simulink model "Australian14gen_R2017a"  (R2017a)
settings: Solver=ode23tb  StartTime=0.0  StopTime=50  FixedStep=1/50  MaxStep=1/50  RelTol=1e-3  AbsTol=1e-1  EnableMultiTasking=on
PreLoadFcn:
  | dataaustralian14gen
values from neighbouring files (symbols this model uses):
  bus_v = [ 101	15 ... (first row only)    [dataaustralian14gen.m]
  comp = [ 1	211	0	0 ... (first row only)    [dataaustralian14gen.m]
  Exc = [ 101	0	 200	0.1	    13.25  2.5	 0	0       0       0       0       0 ... (first row only)    [dataaustralian14gen.m]
  FH = 13    [dataaustralian14gen.m]
  FI = 1    [dataaustralian14gen.m]
  FL = .1    (= 0.1)    [dataaustralian14gen.m]
  G_data = [ 101	333.3	15	3.6	0.14	1.1	0.65	0.25	8.5     0.20	0.05	0       0       0.25	0.2 	0 ... (first row only)    [dataaustralian14gen.m]
  KH = 120    [dataaustralian14gen.m]
  KI = 10    [dataaustralian14gen.m]
  KL = 10    [dataaustralian14gen.m]
  line = [ 102	217	0.0084	0.0667	0.817	330	1 ... (first row only)    [dataaustralian14gen.m]
  p = p_case1    [dataaustralian14gen.m]
  PSSMODEL = 1    [dataaustralian14gen.m]
  SVC = [ 205	650 430   -220 1.055  -68.3 ... (first row only)    [dataaustralian14gen.m]
  trans = [     1   101   102    15   330   333.3    12     12    0.9390 ... (first row only)    [dataaustralian14gen.m]
undefined symbols (not defined in the file or in its folder): D1, Delta
libraries: powerlib x371, sps_avr x14, powerlib_extras x9, factslib x5
(part 2 of 3)

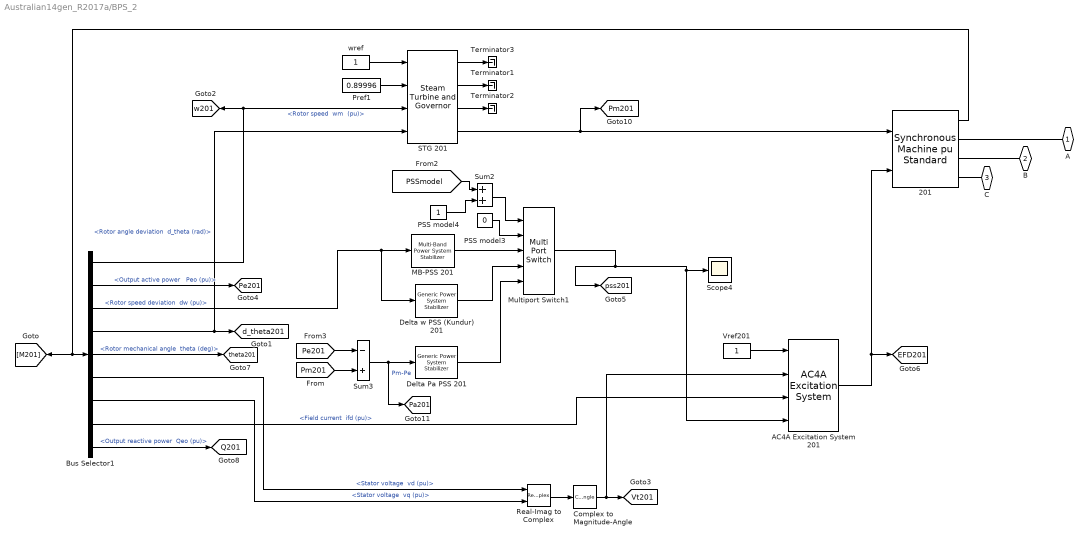
== system Australian14gen_R2017a/BPS_2 ==
  201 : powerlib/Machines/Synchronous Machine pu Standard  PresetModel=No  MechanicalLoad=Mechanical power Pm  ShowDetailedParameters=on  RotorType=Round  Units=per unit standard parameters  MeasurementBus=off  NominalParameters="[G_data(2,2)*1e6  G_data(2,3)*1e3  50]"  Reactances1=[G_data(2,6),G_data(2,8),G_data(2,10),G_data(2,7),G_data(2,12),G_data(2,14),G_data(2,5)]  Reactances2=[G_data(2,6),G_data(2,8),G_data(2,10),G_data(2,7),G_data(2,14),G_data(2,5)]  dAxisTimeConstants=Open-circuit  qAxisTimeConstants=Open-circuit  TimeConstants1="[G_data(2,9)  G_data(2,11)  G_data(2,15)]"  TimeConstants2="[G_data(2,9), G_data(2,11), G_data(2,13),  G_data(2,15)]"  TimeConstants3="[  5.9  0.033  0.023  ]"  TimeConstants4=[ 8.0, 0.03, 0.3371, 0.0295 ]  TimeConstants5=[ 1.01, 0.053, 0.1 ]  TimeConstants6=[ 1.3201, 0.023, 1.0, 0.07 ]  TimeConstants7="[  1.01  0.053  0.051266  ]"  TimeConstants8=[ 1.3201, 0.0231, 0.3371, 0.0295 ]  StatorResistance=0  Mechanical="[ G_data(2,4) 0  4 ]"  PolePairs=4  InitialConditions=[0 9.38697 0.909099 0.909099 0.909099 39.1318 -80.8682 159.132 2.03476]  SetSaturation=off  Saturation=[0.6404,0.7127,0.8441,0.9214,0.9956,1.082,1.19,1.316,1.457;0.7,0.7698,0.8872,0.9466,0.9969,1.046,1.1,1.151,1.201]  LoadFlowParameters=[1 3600000000 20000 0 0]  TsPowergui=0  TsBlock=-1  IterativeModel=Forward Euler  IterativeDiscreteModel=Trapezoidal non iterative  BusType=PV  Pref=p(2,3)*1e6  Qref=0  Qmin=-inf  Qmax=inf  PLF=0  QLF=0
      settings: SourceProductName=Simscape Power Systems
  AC4A Excitation System 201 : sps_avr/AC4A Excitation System  Tr=Exc(2,2)  KaTa="[Exc(2,3)   Exc(2,4)]"  VIminmax=[-10 10]  VRminmax=[-4.53 5.64]  TbTc="[Exc(2,5)  Exc(2,6)]"  Kc=0  v0=[1 2.0348]  TsBlock=0
      settings: SourceProductName=Simscape Power Systems  SourceProductBaseCode=PS
  Bus Selector1 : BusSelector  OutputSignals="Mechanical.Rotor speed  wm  (pu),Output active power   Peo (pu),Mechanical.Rotor speed deviation  dw (pu),Mechanical.Rotor angle deviation  d_theta (rad),Mechanical.Rotor mechanical angle  theta (deg),dq0 components.Stator voltage  vd (pu),dq0 components.Stator voltage  vq (pu),dq0 components.Field current  ifd (pu),Output reactive power  Qeo (pu)"
  Complex to Magnitude-Angle : ComplexToMagnitudeAngle  Output=Magnitude
  Delta Pa PSS 201 : powerlib/Machines/Generic Power System Stabilizer  Tsensor=15e-3  K=2.5*1.25  Twashout=1  Tleadlag1=[60e-3 1]  Tleadlag2=[0 0]  VSlimits=[-0.15 0.15]  Vinit=0  Plot_On=off  MagdB_On=on  FreqRange=logspace(-2,2,500)
      settings: SourceProductName=Simscape Power Systems  SourceProductBaseCode=PS
  Delta w PSS (Kundur) 201 : powerlib/Machines/Generic Power System Stabilizer  Tsensor=15e-3  K=30  Twashout=10  Tleadlag1=[50e-3 20e-3]  Tleadlag2=[3 5.4]  VSlimits=[-0.15 0.15]  Vinit=0  Plot_On=off  MagdB_On=on  FreqRange=logspace(-2,2,500)
      settings: SourceProductName=Simscape Power Systems  SourceProductBaseCode=PS
  MB-PSS 201 : powerlib/Machines/Multi-Band Power System Stabilizer  OperationMode=Simplified settings  Kg=G  GL="[FL  KL]"  GI="[FI  KI]"  GH="[FH  KH]"  GLd=[66 66 9.4]  TcLF=[1.667 2 0 0 0 0 2 2.4 0 0 0 0 1 1]  GId=[66 66 47.6]  TcIF=[1 1 0.25 0.3 0 0 1 1 0.3 0.36 0 0 0 0]  GHd=[66 66 233]  TcHF="[0.01 0.012 0 0 0 0  0.012 0.0144 0 0 0 0 1 1]"  LIM=[.075 .15 .15 .15]  Plot_On=off  MagdB_On=off  FreqRange=logspace(-2,2,500)
      settings: SourceProductName=Simscape Power Systems  SourceProductBaseCode=PS
  Multiport Switch1 : MultiPortSwitch  Inputs=4  InputSameDT=on
  PSS model3 : Constant  Value=0
  PSS model4 : Constant
  Pref1 : Constant  Value=0.89996
  Real-Imag to Complex : RealImagToComplex
  STG 201 : powerlib/Machines/Steam Turbine and Governor  gentype=Tandem-compound (single mass)  reg1="[ 1  0.05    0 ]"  reg2="[ 0.001  0.15 ]"  reg3="[ -0.1  0.1  0  4.496 ]"  N=3000  turb1="[ 0  10   3.3   0.5   ]"  turb2="[   0   0.36    0.36   0.28   ]"  HA="[ 0.046  1.430  1.465   0.192 ]"  KA="[ 90.44  53.88  64.59   62.94  ]"  DA="[ 0.0115  0.3575  0.3663   0.0137  ]"  ini1=0.89996  ini2=[0.779316,-31.4247]
      settings: SourceProductName=Simscape Power Systems  SourceProductBaseCode=PS
  Scope4 : Scope
  Sum2 : Sum  SaturateOnIntegerOverflow=on  InputSameDT=on  OutDataTypeStr=Inherit: Same as first input
  Sum3 : Sum  Inputs=-+  SaturateOnIntegerOverflow=on  InputSameDT=on  OutDataTypeStr=Inherit: Same as first input
  Terminator1 : Terminator
  Terminator2 : Terminator
  Terminator3 : Terminator
  Vref201 : Constant
  wref : Constant
  A : PMIOPort  Port=1  Side=Left
  B : PMIOPort  Port=2  Side=Left
  C : PMIOPort  Port=3  Side=Left
  tag scope: EFD201=global, Pa201=global, Pe201=global, Pm201=global, Q201=global, Vt201=global, d_theta201=global, pss201=global, theta201=global, w201=global
  wires:
  Bus Selector1/7 -> Real-Imag to Complex/2  "<Stator voltage  vq (pu)>"
  Bus Selector1/6 -> Real-Imag to Complex/1  "<Stator voltage  vd (pu)>"
  wref/1 -> STG 201/1
  Vref201/1 -> AC4A Excitation System 201/1
  Bus Selector1/4 -> STG 201/4, [d_theta201]  "<Rotor angle deviation  d_theta (rad)>"
  201/1 -> Bus Selector1/1, [M201]
  Bus Selector1/1 -> [w201], STG 201/3  "<Rotor speed  wm  (pu)>"
  Bus Selector1/3 -> Delta w PSS (Kundur) 201/1, MB-PSS 201/1  "<Rotor speed deviation  dw (pu)>"
  Real-Imag to Complex/1 -> Complex to Magnitude-Angle/1
  Complex to Magnitude-Angle/1 -> AC4A Excitation System 201/2, [Vt201]
  AC4A Excitation System 201/1 -> 201/2, [EFD201]
  Bus Selector1/5 -> [theta201]  "<Rotor mechanical angle  theta (deg)>"
  Bus Selector1/2 -> [Pe201]  "<Output active power   Peo (pu)>"
  Bus Selector1/8 -> AC4A Excitation System 201/3  "<Field current  ifd (pu)>"
  STG 201/4 -> 201/1, [Pm201]
  Bus Selector1/9 -> [Q201]  "<Output reactive power  Qeo (pu)>"
  PSS model4/1 -> Sum2/2
  Sum2/1 -> Multiport Switch1/1
  [PSSmodel] -> Sum2/1
  PSS model3/1 -> Multiport Switch1/2
  Sum3/1 -> [Pa201], Delta Pa PSS 201/1  "Pm-Pe"
  Delta Pa PSS 201/1 -> Multiport Switch1/5
  Delta w PSS (Kundur) 201/1 -> Multiport Switch1/4
  [Pm201] -> Sum3/2
  [Pe201] -> Sum3/1
  MB-PSS 201/1 -> Multiport Switch1/3
  STG 201/1 -> Terminator3/1
  STG 201/2 -> Terminator1/1
  STG 201/3 -> Terminator2/1
  Pref1/1 -> STG 201/2
  Multiport Switch1/1 -> Scope4/1, AC4A Excitation System 201/4, [pss201]
  connections:
  201/RConn1 -- A/RConn1
  201/RConn2 -- B/RConn1
  201/RConn3 -- C/RConn1

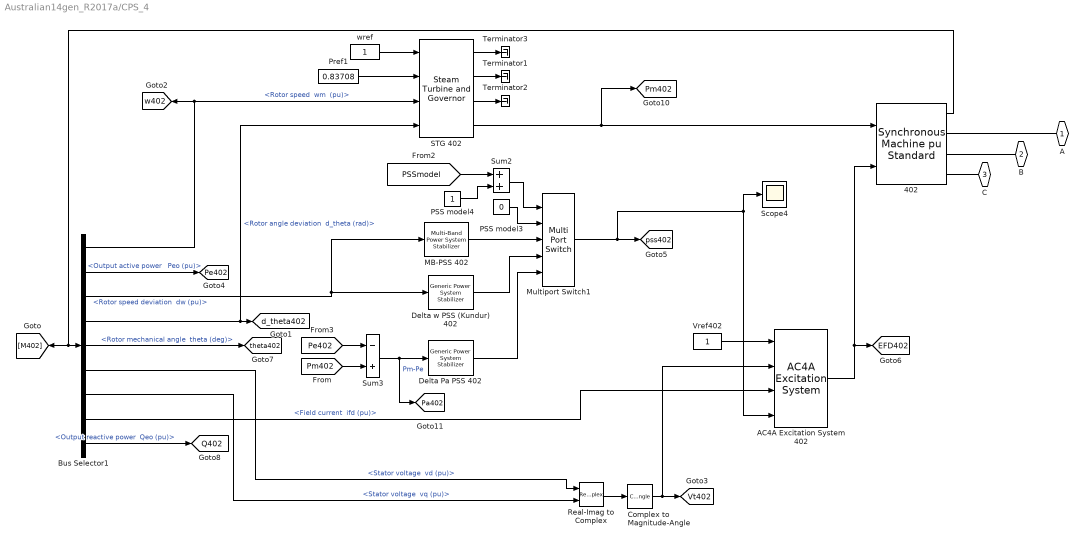
== system Australian14gen_R2017a/CPS_4 ==
  402 : powerlib/Machines/Synchronous Machine pu Standard  PresetModel=No  MechanicalLoad=Mechanical power Pm  ShowDetailedParameters=on  RotorType=Round  Units=per unit standard parameters  MeasurementBus=off  NominalParameters="[G_data(9,2)*1e6  G_data(9,3)*1e3  50]"  Reactances1=[G_data(9,6),G_data(9,8),G_data(9,10),G_data(9,7),G_data(9,12),G_data(9,14),G_data(9,5)]  Reactances2=[G_data(9,6),G_data(9,8),G_data(9,10),G_data(9,7),G_data(9,14),G_data(9,5)]  dAxisTimeConstants=Open-circuit  qAxisTimeConstants=Open-circuit  TimeConstants1="[G_data(9,9)  G_data(9,11)  G_data(9,15)]"  TimeConstants2="[G_data(9,9)  G_data(9,11)  G_data(9,13)  G_data(9,15)]"  TimeConstants3="[  5.9  0.033  0.023  ]"  TimeConstants4=[ 8.0, 0.03, 0.3371, 0.0295 ]  TimeConstants5=[ 1.01, 0.053, 0.1 ]  TimeConstants6=[ 1.3201, 0.023, 1.0, 0.07 ]  TimeConstants7="[  1.01  0.053  0.051266  ]"  TimeConstants8=[ 1.3201, 0.0231, 0.3371, 0.0295 ]  StatorResistance=0  Mechanical="[ G_data(9,4) 0  4 ]"  PolePairs=4  InitialConditions=[0 62.5752 0.854876 0.854876 0.854876 91.9195 -28.0805 211.92 2.07263]  SetSaturation=off  Saturation=[0.6404,0.7127,0.8441,0.9214,0.9956,1.082,1.19,1.316,1.457;0.7,0.7698,0.8872,0.9466,0.9969,1.046,1.1,1.151,1.201]  LoadFlowParameters=[1 837000000 20000 0 0]  TsPowergui=0  TsBlock=-1  IterativeModel=Forward Euler  IterativeDiscreteModel=Trapezoidal non iterative  BusType=PV  Pref=p(9,3)*1e6  Qref=0  Qmin=-inf  Qmax=inf  PLF=0  QLF=0
      settings: SourceProductName=Simscape Power Systems
  AC4A Excitation System 402 : sps_avr/AC4A Excitation System  Tr=Exc(9,2)  KaTa="[Exc(9,3)   Exc(9,4)]"  VIminmax=[-10 10]  VRminmax=[-4.53 5.64]  TbTc="[Exc(9,5)  Exc(9,6)]"  Kc=0  v0=[1 2.0726]  TsBlock=0
      settings: SourceProductName=Simscape Power Systems  SourceProductBaseCode=PS
  Bus Selector1 : BusSelector  OutputSignals="Mechanical.Rotor speed  wm  (pu),Output active power   Peo (pu),Mechanical.Rotor speed deviation  dw (pu),Mechanical.Rotor angle deviation  d_theta (rad),Mechanical.Rotor mechanical angle  theta (deg),dq0 components.Stator voltage  vd (pu),dq0 components.Stator voltage  vq (pu),dq0 components.Field current  ifd (pu),Output reactive power  Qeo (pu)"
  Complex to Magnitude-Angle : ComplexToMagnitudeAngle  Output=Magnitude
  Delta Pa PSS 402 : powerlib/Machines/Generic Power System Stabilizer  Tsensor=15e-3  K=2.5*1.25  Twashout=1  Tleadlag1=[60e-3 1]  Tleadlag2=[0 0]  VSlimits=[-0.15 0.15]  Vinit=0  Plot_On=off  MagdB_On=on  FreqRange=logspace(-2,2,500)
      settings: SourceProductName=Simscape Power Systems  SourceProductBaseCode=PS
  Delta w PSS (Kundur) 402 : powerlib/Machines/Generic Power System Stabilizer  Tsensor=15e-3  K=30  Twashout=10  Tleadlag1=[50e-3 20e-3]  Tleadlag2=[3 5.4]  VSlimits=[-0.15 0.15]  Vinit=0  Plot_On=off  MagdB_On=on  FreqRange=logspace(-2,2,500)
      settings: SourceProductName=Simscape Power Systems  SourceProductBaseCode=PS
  MB-PSS 402 : powerlib/Machines/Multi-Band Power System Stabilizer  OperationMode=Simplified settings  Kg=G  GL="[FL  KL]"  GI="[FI  KI]"  GH="[FH  KH]"  GLd=[66 66 9.4]  TcLF=[1.667 2 0 0 0 0 2 2.4 0 0 0 0 1 1]  GId=[66 66 47.6]  TcIF=[1 1 0.25 0.3 0 0 1 1 0.3 0.36 0 0 0 0]  GHd=[66 66 233]  TcHF="[0.01 0.012 0 0 0 0  0.012 0.0144 0 0 0 0 1 1]"  LIM=[.075 .15 .15 .15]  Plot_On=off  MagdB_On=off  FreqRange=logspace(-2,2,500)
      settings: SourceProductName=Simscape Power Systems  SourceProductBaseCode=PS
  Multiport Switch1 : MultiPortSwitch  Inputs=4  InputSameDT=on
  PSS model3 : Constant  Value=0
  PSS model4 : Constant
  Pref1 : Constant  Value=0.83708
  Real-Imag to Complex : RealImagToComplex
  STG 402 : powerlib/Machines/Steam Turbine and Governor  gentype=Tandem-compound (single mass)  reg1="[ 1  0.05    0 ]"  reg2="[ 0.001  0.15 ]"  reg3="[ -0.1  0.1  0  4.496 ]"  N=3000  turb1="[ 0  10   3.3   0.5   ]"  turb2="[   0   0.36    0.36   0.28   ]"  HA="[ 0.046  1.430  1.465   0.192 ]"  KA="[ 90.44  53.88  64.59   62.94  ]"  DA="[ 0.0115  0.3575  0.3663   0.0137  ]"  ini1=0.83708  ini2=[0.779316,-31.4247]
      settings: SourceProductName=Simscape Power Systems  SourceProductBaseCode=PS
  Scope4 : Scope
  Sum2 : Sum  SaturateOnIntegerOverflow=on  InputSameDT=on  OutDataTypeStr=Inherit: Same as first input
  Sum3 : Sum  Inputs=-+  SaturateOnIntegerOverflow=on  InputSameDT=on  OutDataTypeStr=Inherit: Same as first input
  Terminator1 : Terminator
  Terminator2 : Terminator
  Terminator3 : Terminator
  Vref402 : Constant
  wref : Constant
  A : PMIOPort  Port=1  Side=Left
  B : PMIOPort  Port=2  Side=Left
  C : PMIOPort  Port=3  Side=Left
  tag scope: EFD402=global, Pa402=global, Pe402=global, Pm402=global, Q402=global, Vt402=global, d_theta402=global, pss402=global, theta402=global, w402=global
  wires:
  Bus Selector1/7 -> Real-Imag to Complex/2  "<Stator voltage  vq (pu)>"
  Bus Selector1/6 -> Real-Imag to Complex/1  "<Stator voltage  vd (pu)>"
  wref/1 -> STG 402/1
  Vref402/1 -> AC4A Excitation System 402/1
  Bus Selector1/4 -> STG 402/4, [d_theta402]  "<Rotor angle deviation  d_theta (rad)>"
  402/1 -> Bus Selector1/1, [M402]
  Bus Selector1/1 -> [w402], STG 402/3  "<Rotor speed  wm  (pu)>"
  Bus Selector1/3 -> Delta w PSS (Kundur) 402/1, MB-PSS 402/1  "<Rotor speed deviation  dw (pu)>"
  Real-Imag to Complex/1 -> Complex to Magnitude-Angle/1
  Complex to Magnitude-Angle/1 -> AC4A Excitation System 402/2, [Vt402]
  AC4A Excitation System 402/1 -> 402/2, [EFD402]
  Bus Selector1/5 -> [theta402]  "<Rotor mechanical angle  theta (deg)>"
  Bus Selector1/2 -> [Pe402]  "<Output active power   Peo (pu)>"
  Bus Selector1/8 -> AC4A Excitation System 402/3  "<Field current  ifd (pu)>"
  STG 402/4 -> 402/1, [Pm402]
  Bus Selector1/9 -> [Q402]  "<Output reactive power  Qeo (pu)>"
  PSS model4/1 -> Sum2/2
  Sum2/1 -> Multiport Switch1/1
  [PSSmodel] -> Sum2/1
  PSS model3/1 -> Multiport Switch1/2
  Sum3/1 -> [Pa402], Delta Pa PSS 402/1  "Pm-Pe"
  Delta Pa PSS 402/1 -> Multiport Switch1/5
  Delta w PSS (Kundur) 402/1 -> Multiport Switch1/4
  [Pm402] -> Sum3/2
  [Pe402] -> Sum3/1
  MB-PSS 402/1 -> Multiport Switch1/3
  STG 402/1 -> Terminator3/1
  STG 402/2 -> Terminator1/1
  STG 402/3 -> Terminator2/1
  Pref1/1 -> STG 402/2
  Multiport Switch1/1 -> Scope4/1, AC4A Excitation System 402/4, [pss402]
  connections:
  402/RConn1 -- A/RConn1
  402/RConn2 -- B/RConn1
  402/RConn3 -- C/RConn1

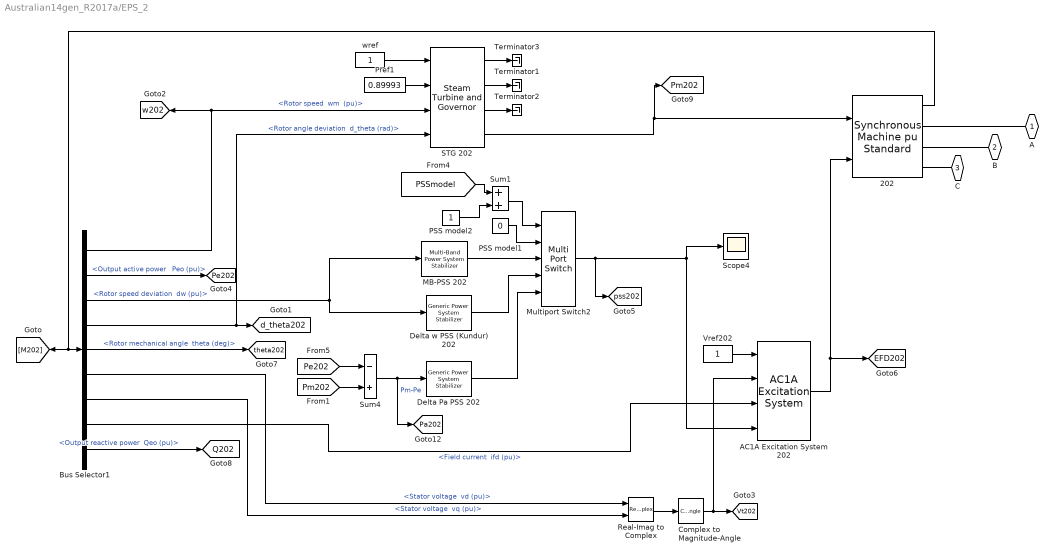
== system Australian14gen_R2017a/EPS_2 ==
  202 : powerlib/Machines/Synchronous Machine pu Standard  PresetModel=No  MechanicalLoad=Mechanical power Pm  ShowDetailedParameters=on  RotorType=Round  Units=per unit standard parameters  MeasurementBus=off  NominalParameters="[G_data(3,2)*1e6  G_data(3,3)*1e3  50]"  Reactances1=[G_data(3,6),G_data(3,8),G_data(3,10),G_data(3,7),G_data(3,12), G_data(3,14),G_data(3,5)]  Reactances2=[G_data(3,6),G_data(3,8),G_data(3,10),G_data(3,7),G_data(3,12), G_data(3,14),G_data(3,5)]  dAxisTimeConstants=Open-circuit  qAxisTimeConstants=Open-circuit  TimeConstants1="[G_data(3,9)  G_data(3,11)  G_data(3,13) G_data(3,15)]"  TimeConstants2="[G_data(3,9)  G_data(3,11)  G_data(3,13) G_data(3,15)]"  TimeConstants3="[  5.9  0.033  0.023  ]"  TimeConstants4=[ 8.0, 0.03, 0.3371, 0.0295 ]  TimeConstants5=[ 1.01, 0.053, 0.1 ]  TimeConstants6=[ 1.3201, 0.023, 1.0, 0.07 ]  TimeConstants7="[  1.01  0.053  0.051266  ]"  TimeConstants8=[ 1.3201, 0.0231, 0.3371, 0.0295 ]  StatorResistance=0  Mechanical="[ G_data(3,4) 0  4 ]"  PolePairs=4  InitialConditions=[0 -1.78632 0.929675 0.929675 0.929675 21.932 -98.068 141.932 2.49164]  SetSaturation=off  Saturation=[0.6404,0.7127,0.8441,0.9214,0.9956,1.082,1.19,1.316,1.457;0.7,0.7698,0.8872,0.9466,0.9969,1.046,1.1,1.151,1.201]  LoadFlowParameters=[1 2500000000 20000 0 0]  TsPowergui=0  TsBlock=-1  IterativeModel=Forward Euler  IterativeDiscreteModel=Trapezoidal non iterative  BusType=PV  Pref=p(3,3)*1e6  Qref=0  Qmin=-inf  Qmax=inf  PLF=0  QLF=0
      settings: SourceProductName=Simscape Power Systems
  AC1A Excitation System 202 : sps_avr/AC1A Excitation System  Tr=Exc(3,2)  KaTa="[Exc(3,3)   Exc(3,4)]"  VAminmax=[-14.5 14.5]  VRminmax=[-5.43 6.03]  KfTf="[Exc(3,9)  Exc(3,10)]"  TbTc="[Exc(3,5)  Exc(3,6)]"  KeTe="[Exc(3,7)  Exc(3,8)]"  Ve12=[4.18 3.14]  SeVe12=[0.10 0.03]  Kd=0.38  Kc=0.20  v0=[1 2.4916]  TsBlock=0
      settings: SourceProductName=Simscape Power Systems  SourceProductBaseCode=PS
  Bus Selector1 : BusSelector  OutputSignals="Mechanical.Rotor speed  wm  (pu),Output active power   Peo (pu),Mechanical.Rotor speed deviation  dw (pu),Mechanical.Rotor angle deviation  d_theta (rad),Mechanical.Rotor mechanical angle  theta (deg),dq0 components.Stator voltage  vd (pu),dq0 components.Stator voltage  vq (pu),dq0 components.Field current  ifd (pu),Output reactive power  Qeo (pu)"
  Complex to Magnitude-Angle : ComplexToMagnitudeAngle  Output=Magnitude
  Delta Pa PSS 202 : powerlib/Machines/Generic Power System Stabilizer  Tsensor=15e-3  K=2.5*1.25  Twashout=1  Tleadlag1=[60e-3 1]  Tleadlag2=[0 0]  VSlimits=[-0.15 0.15]  Vinit=0  Plot_On=off  MagdB_On=on  FreqRange=logspace(-2,2,500)
      settings: SourceProductName=Simscape Power Systems  SourceProductBaseCode=PS
  Delta w PSS (Kundur) 202 : powerlib/Machines/Generic Power System Stabilizer  Tsensor=15e-3  K=30  Twashout=10  Tleadlag1=[50e-3 20e-3]  Tleadlag2=[3 5.4]  VSlimits=[-0.15 0.15]  Vinit=0  Plot_On=off  MagdB_On=on  FreqRange=logspace(-2,2,500)
      settings: SourceProductName=Simscape Power Systems  SourceProductBaseCode=PS
  MB-PSS 202 : powerlib/Machines/Multi-Band Power System Stabilizer  OperationMode=Simplified settings  Kg=G  GL="[FL  KL]"  GI="[FI  KI]"  GH="[FH  KH]"  GLd=[66 66 9.4]  TcLF=[1.667 2 0 0 0 0 2 2.4 0 0 0 0 1 1]  GId=[66 66 47.6]  TcIF=[1 1 0.25 0.3 0 0 1 1 0.3 0.36 0 0 0 0]  GHd=[66 66 233]  TcHF="[0.01 0.012 0 0 0 0  0.012 0.0144 0 0 0 0 1 1]"  LIM=[.075 .15 .15 .15]  Plot_On=off  MagdB_On=off  FreqRange=logspace(-2,2,500)
      settings: SourceProductName=Simscape Power Systems  SourceProductBaseCode=PS
  Multiport Switch2 : MultiPortSwitch  Inputs=4  InputSameDT=on
  PSS model1 : Constant  Value=0
  PSS model2 : Constant
  Pref1 : Constant  Value=0.89993
  Real-Imag to Complex : RealImagToComplex
  STG 202 : powerlib/Machines/Steam Turbine and Governor  gentype=Tandem-compound (single mass)  reg1="[ 1  0.05    0 ]"  reg2="[ 0.001  0.15 ]"  reg3="[ -0.1  0.1  0  4.496 ]"  N=3000  turb1="[ 0  10   3.3   0.5   ]"  turb2="[   0   0.36    0.36   0.28   ]"  HA="[ 0.046  1.430  1.465   0.192 ]"  KA="[ 90.44  53.88  64.59   62.94  ]"  DA="[ 0.0115  0.3575  0.3663   0.0137  ]"  ini1=0.89993  ini2=[0.779316,-31.4247]
      settings: SourceProductName=Simscape Power Systems  SourceProductBaseCode=PS
  Scope4 : Scope
  Sum1 : Sum  SaturateOnIntegerOverflow=on  InputSameDT=on  OutDataTypeStr=Inherit: Same as first input
  Sum4 : Sum  Inputs=-+  SaturateOnIntegerOverflow=on  InputSameDT=on  OutDataTypeStr=Inherit: Same as first input
  Terminator1 : Terminator
  Terminator2 : Terminator
  Terminator3 : Terminator
  Vref202 : Constant
  wref : Constant
  A : PMIOPort  Port=1  Side=Left
  B : PMIOPort  Port=2  Side=Left
  C : PMIOPort  Port=3  Side=Left
  tag scope: EFD202=global, Pa202=global, Pe202=global, Pm202=global, Q202=global, Vt202=global, d_theta202=global, pss202=global, theta202=global, w202=global
  wires:
  Bus Selector1/7 -> Real-Imag to Complex/2  "<Stator voltage  vq (pu)>"
  Bus Selector1/6 -> Real-Imag to Complex/1  "<Stator voltage  vd (pu)>"
  wref/1 -> STG 202/1
  Vref202/1 -> AC1A Excitation System 202/1
  Bus Selector1/4 -> STG 202/4, [d_theta202]  "<Rotor angle deviation  d_theta (rad)>"
  202/1 -> [M202], Bus Selector1/1
  Bus Selector1/1 -> STG 202/3, [w202]  "<Rotor speed  wm  (pu)>"
  Bus Selector1/3 -> MB-PSS 202/1, Delta w PSS (Kundur) 202/1  "<Rotor speed deviation  dw (pu)>"
  Real-Imag to Complex/1 -> Complex to Magnitude-Angle/1
  Complex to Magnitude-Angle/1 -> AC1A Excitation System 202/2, [Vt202]
  AC1A Excitation System 202/1 -> 202/2, [EFD202]
  Bus Selector1/5 -> [theta202]  "<Rotor mechanical angle  theta (deg)>"
  Bus Selector1/2 -> [Pe202]  "<Output active power   Peo (pu)>"
  Bus Selector1/8 -> AC1A Excitation System 202/3  "<Field current  ifd (pu)>"
  STG 202/4 -> 202/1, [Pm202]
  Bus Selector1/9 -> [Q202]  "<Output reactive power  Qeo (pu)>"
  PSS model2/1 -> Sum1/2
  Sum1/1 -> Multiport Switch2/1
  [PSSmodel] -> Sum1/1
  PSS model1/1 -> Multiport Switch2/2
  Sum4/1 -> [Pa202], Delta Pa PSS 202/1  "Pm-Pe"
  Delta Pa PSS 202/1 -> Multiport Switch2/5
  Delta w PSS (Kundur) 202/1 -> Multiport Switch2/4
  [Pm202] -> Sum4/2
  [Pe202] -> Sum4/1
  MB-PSS 202/1 -> Multiport Switch2/3
  STG 202/1 -> Terminator3/1
  STG 202/2 -> Terminator1/1
  STG 202/3 -> Terminator2/1
  Pref1/1 -> STG 202/2
  Multiport Switch2/1 -> Scope4/1, AC1A Excitation System 202/4, [pss202]
  connections:
  202/RConn1 -- A/RConn1
  202/RConn2 -- B/RConn1
  202/RConn3 -- C/RConn1

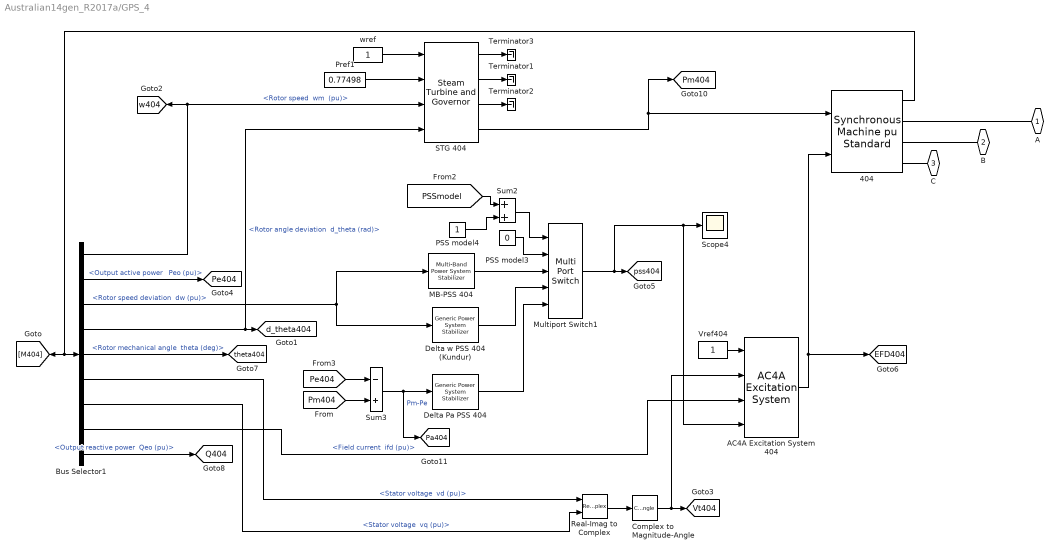
== system Australian14gen_R2017a/GPS_4 ==
  404 : powerlib/Machines/Synchronous Machine pu Standard  PresetModel=No  MechanicalLoad=Mechanical power Pm  ShowDetailedParameters=on  RotorType=Round  Units=per unit standard parameters  MeasurementBus=off  NominalParameters="[G_data(11,2)*1e6  G_data(11,3)*1e3  50]"  Reactances1="[G_data(11,6),G_data(11,8),G_data(11,10),G_data(11,7),  G_data(11,12),G_data(11,14),G_data(11,5)]"  Reactances2="[G_data(11,6),G_data(11,8),G_data(11,10),G_data(11,7),  G_data(11,12),G_data(11,14),G_data(11,5)]"  dAxisTimeConstants=Open-circuit  qAxisTimeConstants=Open-circuit  TimeConstants1="[G_data(11,9)  G_data(11,11)   G_data(11,13) G_data(11,15)]"  TimeConstants2="[G_data(11,9)  G_data(11,11)   G_data(11,13)  G_data(11,15)]"  TimeConstants3="[  5.9  0.033  0.023  ]"  TimeConstants4=[ 8.0, 0.03, 0.3371, 0.0295 ]  TimeConstants5=[ 1.01, 0.053, 0.1 ]  TimeConstants6=[ 1.3201, 0.023, 1.0, 0.07 ]  TimeConstants7="[  1.01  0.053  0.051266  ]"  TimeConstants8=[ 1.3201, 0.0231, 0.3371, 0.0295 ]  StatorResistance=0  Mechanical="[ G_data(11,4) 0  4 ]"  PolePairs=4  InitialConditions=[0 53.761 0.791538 0.791538 0.791538 90.5006 -29.4994 210.501 2.14421]  SetSaturation=off  Saturation=[0.6404,0.7127,0.8441,0.9214,0.9956,1.082,1.19,1.316,1.457;0.7,0.7698,0.8872,0.9466,0.9969,1.046,1.1,1.151,1.201]  LoadFlowParameters=[1 1549800000 20000 0 0]  TsPowergui=0  TsBlock=-1  IterativeModel=Forward Euler  IterativeDiscreteModel=Trapezoidal non iterative  BusType=PV  Pref=p(11,3)*1e6  Qref=0  Qmin=-inf  Qmax=inf  PLF=0  QLF=0
      settings: SourceProductName=Simscape Power Systems
  AC4A Excitation System 404 : sps_avr/AC4A Excitation System  Tr=Exc(11,2)  KaTa="[Exc(11,3)   Exc(11,4)]"  VIminmax=[-10 10]  VRminmax=[-4.53 5.64]  TbTc="[Exc(11,5)  Exc(11,6)]"  Kc=0  v0=[1 2.1442]  TsBlock=0
      settings: SourceProductName=Simscape Power Systems  SourceProductBaseCode=PS
  Bus Selector1 : BusSelector  OutputSignals="Mechanical.Rotor speed  wm  (pu),Output active power   Peo (pu),Mechanical.Rotor speed deviation  dw (pu),Mechanical.Rotor angle deviation  d_theta (rad),Mechanical.Rotor mechanical angle  theta (deg),dq0 components.Stator voltage  vd (pu),dq0 components.Stator voltage  vq (pu),dq0 components.Field current  ifd (pu),Output reactive power  Qeo (pu)"
  Complex to Magnitude-Angle : ComplexToMagnitudeAngle  Output=Magnitude
  "Delta Pa PSS 404 " : powerlib/Machines/Generic Power System Stabilizer  Tsensor=15e-3  K=2.5*1.25  Twashout=1  Tleadlag1=[60e-3 1]  Tleadlag2=[0 0]  VSlimits=[-0.15 0.15]  Vinit=0  Plot_On=off  MagdB_On=on  FreqRange=logspace(-2,2,500)
      settings: SourceProductName=Simscape Power Systems  SourceProductBaseCode=PS
  "Delta w PSS 404 (Kundur) " : powerlib/Machines/Generic Power System Stabilizer  Tsensor=15e-3  K=30  Twashout=10  Tleadlag1=[50e-3 20e-3]  Tleadlag2=[3 5.4]  VSlimits=[-0.15 0.15]  Vinit=0  Plot_On=off  MagdB_On=on  FreqRange=logspace(-2,2,500)
      settings: SourceProductName=Simscape Power Systems  SourceProductBaseCode=PS
  "MB-PSS 404 " : powerlib/Machines/Multi-Band Power System Stabilizer  OperationMode=Simplified settings  Kg=G  GL="[FL  KL]"  GI="[FI  KI]"  GH="[FH  KH]"  GLd=[66 66 9.4]  TcLF=[1.667 2 0 0 0 0 2 2.4 0 0 0 0 1 1]  GId=[66 66 47.6]  TcIF=[1 1 0.25 0.3 0 0 1 1 0.3 0.36 0 0 0 0]  GHd=[66 66 233]  TcHF="[0.01 0.012 0 0 0 0  0.012 0.0144 0 0 0 0 1 1]"  LIM=[.075 .15 .15 .15]  Plot_On=off  MagdB_On=off  FreqRange=logspace(-2,2,500)
      settings: SourceProductName=Simscape Power Systems  SourceProductBaseCode=PS
  Multiport Switch1 : MultiPortSwitch  Inputs=4  InputSameDT=on
  PSS model3 : Constant  Value=0
  PSS model4 : Constant
  Pref1 : Constant  Value=0.77498
  Real-Imag to Complex : RealImagToComplex
  STG 404 : powerlib/Machines/Steam Turbine and Governor  gentype=Tandem-compound (single mass)  reg1="[ 1  0.05    0 ]"  reg2="[ 0.001  0.15 ]"  reg3="[ -0.1  0.1  0  4.496 ]"  N=3000  turb1="[ 0  10   3.3   0.5   ]"  turb2="[   0   0.36    0.36   0.28   ]"  HA="[ 0.046  1.430  1.465   0.192 ]"  KA="[ 90.44  53.88  64.59   62.94  ]"  DA="[ 0.0115  0.3575  0.3663   0.0137  ]"  ini1=0.77498  ini2=[0.779316,-31.4247]
      settings: SourceProductName=Simscape Power Systems  SourceProductBaseCode=PS
  Scope4 : Scope
  Sum2 : Sum  SaturateOnIntegerOverflow=on  InputSameDT=on  OutDataTypeStr=Inherit: Same as first input
  Sum3 : Sum  Inputs=-+  SaturateOnIntegerOverflow=on  InputSameDT=on  OutDataTypeStr=Inherit: Same as first input
  Terminator1 : Terminator
  Terminator2 : Terminator
  Terminator3 : Terminator
  Vref404 : Constant
  wref : Constant
  A : PMIOPort  Port=1  Side=Left
  B : PMIOPort  Port=2  Side=Left
  C : PMIOPort  Port=3  Side=Left
  tag scope: EFD404=global, Pa404=global, Pe404=global, Pm404=global, Q404=global, Vt404=global, d_theta404=global, pss404=global, theta404=global, w404=global
  wires:
  Bus Selector1/7 -> Real-Imag to Complex/2  "<Stator voltage  vq (pu)>"
  Bus Selector1/6 -> Real-Imag to Complex/1  "<Stator voltage  vd (pu)>"
  wref/1 -> STG 404/1
  Vref404/1 -> AC4A Excitation System 404/1
  Bus Selector1/4 -> STG 404/4, [d_theta404]  "<Rotor angle deviation  d_theta (rad)>"
  404/1 -> [M404], Bus Selector1/1
  Bus Selector1/1 -> [w404], STG 404/3  "<Rotor speed  wm  (pu)>"
  Bus Selector1/3 -> "MB-PSS 404 "/1, "Delta w PSS 404 (Kundur) "/1  "<Rotor speed deviation  dw (pu)>"
  Real-Imag to Complex/1 -> Complex to Magnitude-Angle/1
  Complex to Magnitude-Angle/1 -> AC4A Excitation System 404/2, [Vt404]
  AC4A Excitation System 404/1 -> 404/2, [EFD404]
  Bus Selector1/5 -> [theta404]  "<Rotor mechanical angle  theta (deg)>"
  Bus Selector1/2 -> [Pe404]  "<Output active power   Peo (pu)>"
  Bus Selector1/8 -> AC4A Excitation System 404/3  "<Field current  ifd (pu)>"
  STG 404/4 -> 404/1, [Pm404]
  Bus Selector1/9 -> [Q404]  "<Output reactive power  Qeo (pu)>"
  PSS model4/1 -> Sum2/2
  Sum2/1 -> Multiport Switch1/1
  [PSSmodel] -> Sum2/1
  PSS model3/1 -> Multiport Switch1/2
  Sum3/1 -> [Pa404], "Delta Pa PSS 404 "/1  "Pm-Pe"
  "Delta Pa PSS 404 "/1 -> Multiport Switch1/5
  "Delta w PSS 404 (Kundur) "/1 -> Multiport Switch1/4
  [Pm404] -> Sum3/2
  [Pe404] -> Sum3/1
  "MB-PSS 404 "/1 -> Multiport Switch1/3
  STG 404/1 -> Terminator3/1
  STG 404/2 -> Terminator1/1
  STG 404/3 -> Terminator2/1
  Pref1/1 -> STG 404/2
  Multiport Switch1/1 -> AC4A Excitation System 404/4, Scope4/1, [pss404]
  connections:
  404/RConn1 -- A/RConn1
  404/RConn2 -- B/RConn1
  404/RConn3 -- C/RConn1

== system Australian14gen_R2017a/HPS_1 ==
  101 : powerlib/Machines/Synchronous Machine pu Standard  PresetModel=No  MechanicalLoad=Mechanical power Pm  ShowDetailedParameters=on  RotorType=Salient-pole  Units=per unit standard parameters  MeasurementBus=off  NominalParameters="[G_data(1,2)*1e6  G_data(1,3)*1e3  50]"  Reactances1="[G_data(1,6),G_data(1,8),G_data(1,10),G_data(1,7),  G_data(1,12),G_data(1,14),G_data(1,5)]"  Reactances2=[G_data(1,6),G_data(1,8),G_data(1,10),G_data(1,7),G_data(1,14),G_data(1,5)]  dAxisTimeConstants=Open-circuit  qAxisTimeConstants=Open-circuit  TimeConstants1="[G_data(1,9)  G_data(1,11)  G_data(1,15)]"  TimeConstants2="[G_data(1,9)  G_data(1,11)   G_data(1,13)  G_data(1,15)]"  TimeConstants3="[  5.9  0.033  0.023  ]"  TimeConstants4="[G_data(1,9)  G_data(1,11)   G_data(1,13)  G_data(1,15)]"  TimeConstants5=[ 1.01, 0.053, 0.1 ]  TimeConstants6=[ 1.3201, 0.023, 1.0, 0.07 ]  TimeConstants7="[  1.01  0.053  0.051266  ]"  TimeConstants8=[ 1.3201, 0.0231, 0.3371, 0.0295 ]  StatorResistance=0  Mechanical="[ G_data(1,4) 0  4 ]"  PolePairs=4  InitialConditions=[0 -80.9796 0.362751 0.362751 0.362751 -39.3016 -159.302 80.6984 1.28566]  SetSaturation=off  Saturation=[0.6404,0.7127,0.8441,0.9214,0.9956,1.082,1.19,1.316,1.457;0.7,0.7698,0.8872,0.9466,0.9969,1.046,1.1,1.151,1.201]  LoadFlowParameters=[2 370000000 15000 0 0]  TsPowergui=0  TsBlock=-1  IterativeModel=Forward Euler  IterativeDiscreteModel=Trapezoidal non iterative  BusType=swing  Pref=p(1,3)*1e6  Qref=0  Qmin=-inf  Qmax=inf  PLF=0  QLF=0
      settings: SourceProductName=Simscape Power Systems
  AC4A Excitation System 101 : sps_avr/AC4A Excitation System  Tr=Exc(1,2)  KaTa="[Exc(1,3)   Exc(1,4)]"  VIminmax=[-10 10]  VRminmax=[-4.53 5.64]  TbTc="[Exc(1,5)  Exc(1,6)]"  Kc=0  v0=[1 1.2857]  TsBlock=0
      settings: SourceProductName=Simscape Power Systems  SourceProductBaseCode=PS
  Bus Selector1 : BusSelector  OutputSignals="Mechanical.Rotor speed  wm  (pu),Output active power   Peo (pu),Mechanical.Rotor speed deviation  dw (pu),Mechanical.Rotor angle deviation  d_theta (rad),Mechanical.Rotor mechanical angle  theta (deg),dq0 components.Stator voltage  vd (pu),dq0 components.Stator voltage  vq (pu),dq0 components.Field current  ifd (pu),Output reactive power  Qeo (pu)"
  Complex to Magnitude-Angle : ComplexToMagnitudeAngle  Output=Magnitude
  Delta Pa PSS  101 : powerlib/Machines/Generic Power System Stabilizer  Tsensor=15e-3  K=2.5*1.25  Twashout=1  Tleadlag1=[60e-3 1]  Tleadlag2=[0 0]  VSlimits=[-0.15 0.15]  Vinit=0  Plot_On=off  MagdB_On=on  FreqRange=logspace(-2,2,500)
      settings: SourceProductName=Simscape Power Systems  SourceProductBaseCode=PS
  Delta w PSS (Kundur)  101 : powerlib/Machines/Generic Power System Stabilizer  Tsensor=15e-3  K=30  Twashout=10  Tleadlag1=[50e-3 20e-3]  Tleadlag2=[3 5.4]  VSlimits=[-0.15 0.15]  Vinit=0  Plot_On=off  MagdB_On=on  FreqRange=logspace(-2,2,500)
      settings: SourceProductName=Simscape Power Systems  SourceProductBaseCode=PS
  MB-PSS  101 : powerlib/Machines/Multi-Band Power System Stabilizer  OperationMode=Simplified settings  Kg=G  GL="[FL  KL]"  GI="[FI  KI]"  GH="[FH  KH]"  GLd=[66 66 9.4]  TcLF=[1.667 2 0 0 0 0 2 2.4 0 0 0 0 1 1]  GId=[66 66 47.6]  TcIF=[1 1 0.25 0.3 0 0 1 1 0.3 0.36 0 0 0 0]  GHd=[66 66 233]  TcHF="[0.01 0.012 0 0 0 0  0.012 0.0144 0 0 0 0 1 1]"  LIM=[.075 .15 .15 .15]  Plot_On=off  MagdB_On=off  FreqRange=logspace(-2,2,500)
      settings: SourceProductName=Simscape Power Systems  SourceProductBaseCode=PS
  Multiport Switch1 : MultiPortSwitch  Inputs=4  InputSameDT=on
  PSS model3 : Constant  Value=0
  PSS model4 : Constant
  Pref : Constant  Value=0.306
  Real-Imag to Complex : RealImagToComplex
  Scope4 : Scope
  Sum2 : Sum  SaturateOnIntegerOverflow=on  InputSameDT=on  OutDataTypeStr=Inherit: Same as first input
  Sum3 : Sum  Inputs=-+  SaturateOnIntegerOverflow=on  InputSameDT=on  OutDataTypeStr=Inherit: Same as first input
  Vref101 : Constant
  A : PMIOPort  Port=1  Side=Left
  B : PMIOPort  Port=2  Side=Left
  C : PMIOPort  Port=3  Side=Left
  tag scope: EFD101=global, Pa101=global, Pe101=global, Pm101=global, Q101=global, Vt101=global, d_theta101=global, pss101=global, theta101=global, w101=global
  wires:
  Bus Selector1/7 -> Real-Imag to Complex/2  "<Stator voltage  vq (pu)>"
  Bus Selector1/6 -> Real-Imag to Complex/1  "<Stator voltage  vd (pu)>"
  Vref101/1 -> AC4A Excitation System 101/1
  Bus Selector1/4 -> [d_theta101]  "<Rotor angle deviation  d_theta (rad)>"
  101/1 -> Bus Selector1/1, [M101]
  Bus Selector1/1 -> [w101]  "<Rotor speed  wm  (pu)>"
  Bus Selector1/3 -> Delta w PSS (Kundur)  101/1, MB-PSS  101/1  "<Rotor speed deviation  dw (pu)>"
  Real-Imag to Complex/1 -> Complex to Magnitude-Angle/1
  AC4A Excitation System 101/1 -> 101/2, [EFD101]
  Bus Selector1/5 -> [theta101]  "<Rotor mechanical angle  theta (deg)>"
  Bus Selector1/2 -> [Pe101]  "<Output active power   Peo (pu)>"
  Bus Selector1/8 -> AC4A Excitation System 101/3  "<Field current  ifd (pu)>"
  Complex to Magnitude-Angle/1 -> AC4A Excitation System 101/2, [Vt101]
  Pref/1 -> [Pm101], 101/1
  Bus Selector1/9 -> [Q101]  "<Output reactive power  Qeo (pu)>"
  PSS model4/1 -> Sum2/2
  Sum2/1 -> Multiport Switch1/1
  [PSSmodel] -> Sum2/1
  PSS model3/1 -> Multiport Switch1/2
  Sum3/1 -> [Pa101], Delta Pa PSS  101/1  "Pm-Pe"
  Delta Pa PSS  101/1 -> Multiport Switch1/5
  Delta w PSS (Kundur)  101/1 -> Multiport Switch1/4
  [Pm101] -> Sum3/2
  [Pe101] -> Sum3/1
  MB-PSS  101/1 -> Multiport Switch1/3
  Multiport Switch1/1 -> AC4A Excitation System 101/4, Scope4/1, [pss101]
  connections:
  101/RConn1 -- A/RConn1
  101/RConn2 -- B/RConn1
  101/RConn3 -- C/RConn1

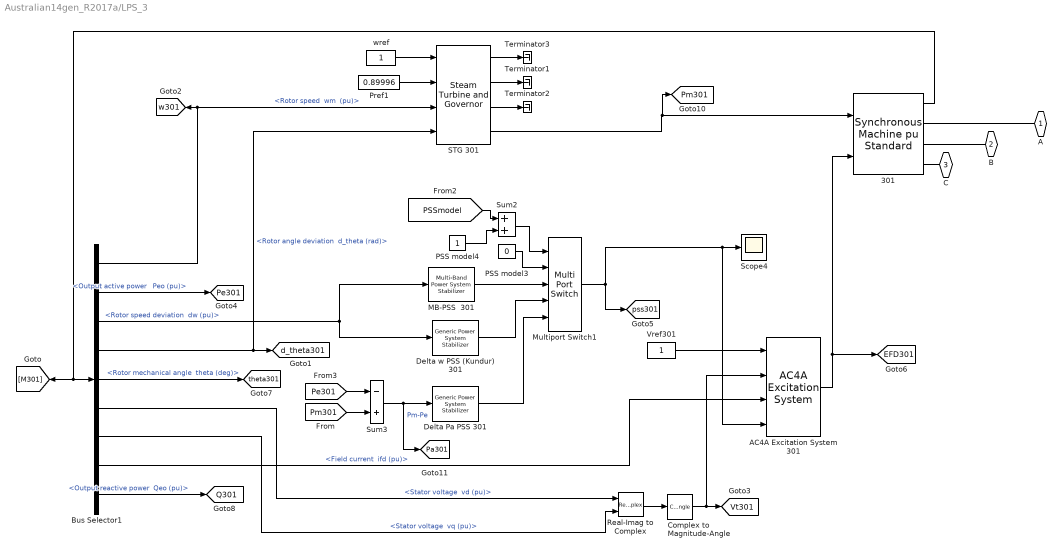
== system Australian14gen_R2017a/LPS_3 ==
  301 : powerlib/Machines/Synchronous Machine pu Standard  PresetModel=No  MechanicalLoad=Mechanical power Pm  ShowDetailedParameters=on  RotorType=Round  Units=per unit standard parameters  MeasurementBus=off  NominalParameters="[G_data(6,2)*1E6  G_data(6,3)*1E3  50]"  Reactances1=[G_data(6,6),G_data(6,8),G_data(6,10),G_data(6,7),G_data(6,12),G_data(6,14),G_data(6,5)]  Reactances2=[G_data(6,6),G_data(6,8),G_data(6,10),G_data(6,7),G_data(6,12),G_data(6,14),G_data(6,5)]  dAxisTimeConstants=Open-circuit  qAxisTimeConstants=Open-circuit  TimeConstants1="[G_data(6,9)  G_data(6,11)  G_data(6,13)  G_data(6,15)]"  TimeConstants2="[G_data(6,9)  G_data(6,11)  G_data(6,13)  G_data(6,15)]"  TimeConstants3="[  5.9  0.033  0.023  ]"  TimeConstants4=[ 8.0, 0.03, 0.3371, 0.0295 ]  TimeConstants5=[ 1.01, 0.053, 0.1 ]  TimeConstants6=[ 1.3201, 0.023, 1.0, 0.07 ]  TimeConstants7="[  1.01  0.053  0.051266  ]"  TimeConstants8=[ 1.3201, 0.0231, 0.3371, 0.0295 ]  StatorResistance=0  Mechanical="[ G_data(6,4) 0  4 ]"  PolePairs=4  InitialConditions=[0 -49.2714 0.929226 0.929226 0.929226 -18.7511 -138.751 101.249 2.86766]  SetSaturation=off  Saturation=[0.6404,0.7127,0.8441,0.9214,0.9956,1.082,1.19,1.316,1.457;0.7,0.7698,0.8872,0.9466,0.9969,1.046,1.1,1.151,1.201]  LoadFlowParameters=[1 4200000000 20000 0 0]  TsPowergui=0  TsBlock=-1  IterativeModel=Forward Euler  IterativeDiscreteModel=Trapezoidal non iterative  BusType=PV  Pref=p(6,3)*1e6  Qref=0  Qmin=-inf  Qmax=inf  PLF=0  QLF=0
      settings: SourceProductName=Simscape Power Systems
  AC4A Excitation System 301 : sps_avr/AC4A Excitation System  Tr=Exc(6,2)  KaTa="[Exc(6,3)   Exc(6,4)]"  VIminmax=[-10 10]  VRminmax=[-4.53 5.64]  TbTc="[Exc(6,5)  Exc(6,6)]"  Kc=0  v0=[1 2.8677]  TsBlock=0
      settings: SourceProductName=Simscape Power Systems  SourceProductBaseCode=PS
  Bus Selector1 : BusSelector  OutputSignals="Mechanical.Rotor speed  wm  (pu),Output active power   Peo (pu),Mechanical.Rotor speed deviation  dw (pu),Mechanical.Rotor angle deviation  d_theta (rad),Mechanical.Rotor mechanical angle  theta (deg),dq0 components.Stator voltage  vd (pu),dq0 components.Stator voltage  vq (pu),dq0 components.Field current  ifd (pu),Output reactive power  Qeo (pu)"
  Complex to Magnitude-Angle : ComplexToMagnitudeAngle  Output=Magnitude
  "Delta Pa PSS 301 " : powerlib/Machines/Generic Power System Stabilizer  Tsensor=15e-3  K=2.5*1.25  Twashout=1  Tleadlag1=[60e-3 1]  Tleadlag2=[0 0]  VSlimits=[-0.15 0.15]  Vinit=0  Plot_On=off  MagdB_On=on  FreqRange=logspace(-2,2,500)
      settings: SourceProductName=Simscape Power Systems  SourceProductBaseCode=PS
  "Delta w PSS (Kundur) 301 " : powerlib/Machines/Generic Power System Stabilizer  Tsensor=15e-3  K=30  Twashout=10  Tleadlag1=[50e-3 20e-3]  Tleadlag2=[3 5.4]  VSlimits=[-0.15 0.15]  Vinit=0  Plot_On=off  MagdB_On=on  FreqRange=logspace(-2,2,500)
      settings: SourceProductName=Simscape Power Systems  SourceProductBaseCode=PS
  MB-PSS  301 : powerlib/Machines/Multi-Band Power System Stabilizer  OperationMode=Simplified settings  Kg=G  GL="[FL  KL]"  GI="[FI  KI]"  GH="[FH  KH]"  GLd=[66 66 9.4]  TcLF=[1.667 2 0 0 0 0 2 2.4 0 0 0 0 1 1]  GId=[66 66 47.6]  TcIF=[1 1 0.25 0.3 0 0 1 1 0.3 0.36 0 0 0 0]  GHd=[66 66 233]  TcHF="[0.01 0.012 0 0 0 0  0.012 0.0144 0 0 0 0 1 1]"  LIM=[.075 .15 .15 .15]  Plot_On=off  MagdB_On=off  FreqRange=logspace(-2,2,500)
      settings: SourceProductName=Simscape Power Systems  SourceProductBaseCode=PS
  Multiport Switch1 : MultiPortSwitch  Inputs=4  InputSameDT=on
  PSS model3 : Constant  Value=0
  PSS model4 : Constant
  Pref1 : Constant  Value=0.89996
  Real-Imag to Complex : RealImagToComplex
  STG 301 : powerlib/Machines/Steam Turbine and Governor  gentype=Tandem-compound (single mass)  reg1="[ 1  0.05    0 ]"  reg2="[ 0.001  0.15 ]"  reg3="[ -0.1  0.1  0  4.496 ]"  N=3000  turb1="[ 0  10   3.3   0.5   ]"  turb2="[   0   0.36    0.36   0.28   ]"  HA="[ 0.046  1.430  1.465   0.192 ]"  KA="[ 90.44  53.88  64.59   62.94  ]"  DA="[ 0.0115  0.3575  0.3663   0.0137  ]"  ini1=0.89996  ini2=[0.779316,-31.4247]
      settings: SourceProductName=Simscape Power Systems  SourceProductBaseCode=PS
  Scope4 : Scope
  Sum2 : Sum  SaturateOnIntegerOverflow=on  InputSameDT=on  OutDataTypeStr=Inherit: Same as first input
  Sum3 : Sum  Inputs=-+  SaturateOnIntegerOverflow=on  InputSameDT=on  OutDataTypeStr=Inherit: Same as first input
  Terminator1 : Terminator
  Terminator2 : Terminator
  Terminator3 : Terminator
  Vref301 : Constant
  wref : Constant
  A : PMIOPort  Port=1  Side=Left
  B : PMIOPort  Port=2  Side=Left
  C : PMIOPort  Port=3  Side=Left
  tag scope: EFD301=global, Pa301=global, Pe301=global, Pm301=global, Q301=global, Vt301=global, d_theta301=global, pss301=global, theta301=global, w301=global
  wires:
  Bus Selector1/7 -> Real-Imag to Complex/2  "<Stator voltage  vq (pu)>"
  Bus Selector1/6 -> Real-Imag to Complex/1  "<Stator voltage  vd (pu)>"
  wref/1 -> STG 301/1
  Vref301/1 -> AC4A Excitation System 301/1
  Bus Selector1/4 -> [d_theta301], STG 301/4  "<Rotor angle deviation  d_theta (rad)>"
  301/1 -> Bus Selector1/1, [M301]
  Bus Selector1/1 -> [w301], STG 301/3  "<Rotor speed  wm  (pu)>"
  Bus Selector1/3 -> "Delta w PSS (Kundur) 301 "/1, MB-PSS  301/1  "<Rotor speed deviation  dw (pu)>"
  Real-Imag to Complex/1 -> Complex to Magnitude-Angle/1
  Complex to Magnitude-Angle/1 -> AC4A Excitation System 301/2, [Vt301]
  AC4A Excitation System 301/1 -> 301/2, [EFD301]
  Bus Selector1/5 -> [theta301]  "<Rotor mechanical angle  theta (deg)>"
  Bus Selector1/2 -> [Pe301]  "<Output active power   Peo (pu)>"
  Bus Selector1/8 -> AC4A Excitation System 301/3  "<Field current  ifd (pu)>"
  STG 301/4 -> 301/1, [Pm301]
  Bus Selector1/9 -> [Q301]  "<Output reactive power  Qeo (pu)>"
  PSS model4/1 -> Sum2/2
  Sum2/1 -> Multiport Switch1/1
  [PSSmodel] -> Sum2/1
  PSS model3/1 -> Multiport Switch1/2
  Sum3/1 -> [Pa301], "Delta Pa PSS 301 "/1  "Pm-Pe"
  "Delta Pa PSS 301 "/1 -> Multiport Switch1/5
  "Delta w PSS (Kundur) 301 "/1 -> Multiport Switch1/4
  [Pm301] -> Sum3/2
  [Pe301] -> Sum3/1
  MB-PSS  301/1 -> Multiport Switch1/3
  STG 301/1 -> Terminator3/1
  STG 301/2 -> Terminator1/1
  STG 301/3 -> Terminator2/1
  Pref1/1 -> STG 301/2
  Multiport Switch1/1 -> Scope4/1, AC4A Excitation System 301/4, [pss301]
  connections:
  301/RConn1 -- A/RConn1
  301/RConn2 -- B/RConn1
  301/RConn3 -- C/RConn1

== system Australian14gen_R2017a/MEASUREMENTS ==
  Add : Sum  Inputs=+-
  Add1 : Sum
  Constant : Constant
  Constant1 : Constant  Value=50
  Gain : Gain  Gain=1/14
  Gain1 : Gain  Gain=50
  Mean Frequency : Scope
  Mux4 : Mux  Inputs=14
  Sum of Elements : Sum  Inputs=+
  W14 : ToWorkspace  VariableName=W  SaveFormat=Structure With Time  SampleTime=1/50
  W5 : ToWorkspace  VariableName=Fr  SaveFormat=Structure With Time  SampleTime=1/50
  wires:
  [w101] -> Mux4/1
  [w201] -> Mux4/2
  [w202] -> Mux4/3
  [w203] -> Mux4/4
  [w204] -> Mux4/5
  [w301] -> Mux4/6
  [w302] -> Mux4/7
  [w401] -> Mux4/8
  [w402] -> Mux4/9
  [w503] -> Mux4/14
  [w502] -> Mux4/13
  [w501] -> Mux4/12
  [w401] -> Mux4/10
  [w401] -> Mux4/11
  Mux4/1 -> Sum of Elements/1, W14/1
  Sum of Elements/1 -> Gain/1
  Constant/1 -> Add/2
  Gain/1 -> Add/1
  Constant1/1 -> Add1/2
  Gain1/1 -> Add1/1
  Add/1 -> Gain1/1
  Add1/1 -> Mean Frequency/1, W5/1  "Mean frequency (Hz)"

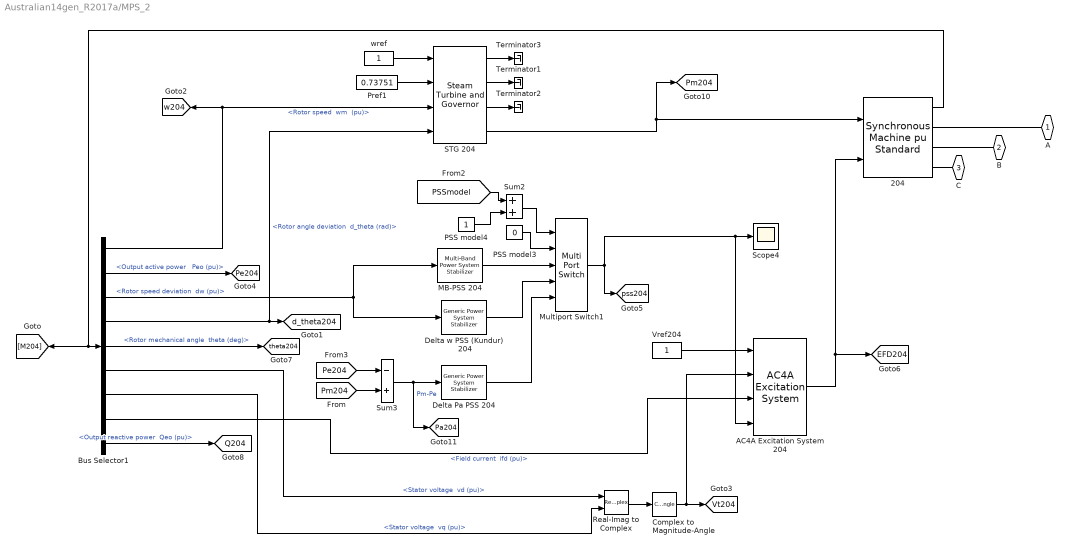
== system Australian14gen_R2017a/MPS_2 ==
  204 : powerlib/Machines/Synchronous Machine pu Standard  PresetModel=No  MechanicalLoad=Mechanical power Pm  ShowDetailedParameters=on  RotorType=Round  Units=per unit standard parameters  MeasurementBus=off  NominalParameters="[G_data(5,2)*1E6  G_data(5,3)*1E3  50]"  Reactances1=[G_data(5,6),G_data(5,8),G_data(5,10),G_data(5,7),G_data(5,12),G_data(5,14),G_data(5,5)]  Reactances2=[G_data(5,6),G_data(5,8),G_data(5,10),G_data(5,7),G_data(5,12),G_data(5,14),G_data(5,5)]  dAxisTimeConstants=Open-circuit  qAxisTimeConstants=Open-circuit  TimeConstants1="[G_data(5,9)  G_data(5,11)  G_data(5,13) G_data(5,15)]"  TimeConstants2="[G_data(5,9)  G_data(5,11)  G_data(5,13) G_data(5,15)]"  TimeConstants3="[  5.9  0.033  0.023  ]"  TimeConstants4=[ 8.0, 0.03, 0.3371, 0.0295 ]  TimeConstants5=[ 1.01, 0.053, 0.1 ]  TimeConstants6=[ 1.3201, 0.023, 1.0, 0.07 ]  TimeConstants7="[  1.01  0.053  0.051266  ]"  TimeConstants8=[ 1.3201, 0.0231, 0.3371, 0.0295 ]  StatorResistance=0  Mechanical="[ G_data(5,4) 0  4 ]"  PolePairs=4  InitialConditions=[0 -7.58215 0.758362 0.758362 0.758362 24.3574 -95.6426 144.357 1.87049]  SetSaturation=off  Saturation=[0.6404,0.7127,0.8441,0.9214,0.9956,1.082,1.19,1.316,1.457;0.7,0.7698,0.8872,0.9466,0.9969,1.046,1.1,1.151,1.201]  LoadFlowParameters=[1 2950200000 20000 0 0]  TsPowergui=0  TsBlock=-1  IterativeModel=Forward Euler  IterativeDiscreteModel=Trapezoidal non iterative  BusType=PV  Pref=p(5,3)*1e6  Qref=0  Qmin=-inf  Qmax=inf  PLF=0  QLF=0
      settings: SourceProductName=Simscape Power Systems
  AC4A Excitation System 204 : sps_avr/AC4A Excitation System  Tr=Exc(5,2)  KaTa="[Exc(5,3)   Exc(5,4)]"  VIminmax=[-10 10]  VRminmax=[-4.53 5.64]  TbTc="[Exc(5,5)  Exc(5,6)]"  Kc=0  v0=[1 1.8705]  TsBlock=0
      settings: SourceProductName=Simscape Power Systems  SourceProductBaseCode=PS
  Bus Selector1 : BusSelector  OutputSignals="Mechanical.Rotor speed  wm  (pu),Output active power   Peo (pu),Mechanical.Rotor speed deviation  dw (pu),Mechanical.Rotor angle deviation  d_theta (rad),Mechanical.Rotor mechanical angle  theta (deg),dq0 components.Stator voltage  vd (pu),dq0 components.Stator voltage  vq (pu),dq0 components.Field current  ifd (pu),Output reactive power  Qeo (pu)"
  Complex to Magnitude-Angle : ComplexToMagnitudeAngle  Output=Magnitude
  "Delta Pa PSS 204 " : powerlib/Machines/Generic Power System Stabilizer  Tsensor=15e-3  K=2.5*1.25  Twashout=1  Tleadlag1=[60e-3 1]  Tleadlag2=[0 0]  VSlimits=[-0.15 0.15]  Vinit=0  Plot_On=off  MagdB_On=on  FreqRange=logspace(-2,2,500)
      settings: SourceProductName=Simscape Power Systems  SourceProductBaseCode=PS
  Delta w PSS (Kundur)  204 : powerlib/Machines/Generic Power System Stabilizer  Tsensor=15e-3  K=30  Twashout=10  Tleadlag1=[50e-3 20e-3]  Tleadlag2=[3 5.4]  VSlimits=[-0.15 0.15]  Vinit=0  Plot_On=off  MagdB_On=on  FreqRange=logspace(-2,2,500)
      settings: SourceProductName=Simscape Power Systems  SourceProductBaseCode=PS
  "MB-PSS 204 " : powerlib/Machines/Multi-Band Power System Stabilizer  OperationMode=Simplified settings  Kg=G  GL="[FL  KL]"  GI="[FI  KI]"  GH="[FH  KH]"  GLd=[66 66 9.4]  TcLF=[1.667 2 0 0 0 0 2 2.4 0 0 0 0 1 1]  GId=[66 66 47.6]  TcIF=[1 1 0.25 0.3 0 0 1 1 0.3 0.36 0 0 0 0]  GHd=[66 66 233]  TcHF="[0.01 0.012 0 0 0 0  0.012 0.0144 0 0 0 0 1 1]"  LIM=[.075 .15 .15 .15]  Plot_On=off  MagdB_On=off  FreqRange=logspace(-2,2,500)
      settings: SourceProductName=Simscape Power Systems  SourceProductBaseCode=PS
  Multiport Switch1 : MultiPortSwitch  Inputs=4  InputSameDT=on
  PSS model3 : Constant  Value=0
  PSS model4 : Constant
  Pref1 : Constant  Value=0.73751
  Real-Imag to Complex : RealImagToComplex
  STG 204 : powerlib/Machines/Steam Turbine and Governor  gentype=Tandem-compound (single mass)  reg1="[ 1  0.05    0 ]"  reg2="[ 0.001  0.15 ]"  reg3="[ -0.1  0.1  0  4.496 ]"  N=3000  turb1="[ 0  10   3.3   0.5   ]"  turb2="[   0   0.36    0.36   0.28   ]"  HA="[ 0.046  1.430  1.465   0.192 ]"  KA="[ 90.44  53.88  64.59   62.94  ]"  DA="[ 0.0115  0.3575  0.3663   0.0137  ]"  ini1=0.73751  ini2=[0.779316,-31.4247]
      settings: SourceProductName=Simscape Power Systems  SourceProductBaseCode=PS
  Scope4 : Scope
  Sum2 : Sum  SaturateOnIntegerOverflow=on  InputSameDT=on  OutDataTypeStr=Inherit: Same as first input
  Sum3 : Sum  Inputs=-+  SaturateOnIntegerOverflow=on  InputSameDT=on  OutDataTypeStr=Inherit: Same as first input
  Terminator1 : Terminator
  Terminator2 : Terminator
  Terminator3 : Terminator
  Vref204 : Constant
  wref : Constant
  A : PMIOPort  Port=1  Side=Left
  B : PMIOPort  Port=2  Side=Left
  C : PMIOPort  Port=3  Side=Left
  tag scope: EFD204=global, Pa204=global, Pe204=global, Pm204=global, Q204=global, Vt204=global, d_theta204=global, pss204=global, theta204=global, w204=global
  wires:
  Bus Selector1/7 -> Real-Imag to Complex/2  "<Stator voltage  vq (pu)>"
  Bus Selector1/6 -> Real-Imag to Complex/1  "<Stator voltage  vd (pu)>"
  wref/1 -> STG 204/1
  Vref204/1 -> AC4A Excitation System 204/1
  Bus Selector1/4 -> STG 204/4, [d_theta204]  "<Rotor angle deviation  d_theta (rad)>"
  204/1 -> [M204], Bus Selector1/1
  Bus Selector1/1 -> [w204], STG 204/3  "<Rotor speed  wm  (pu)>"
  Bus Selector1/3 -> Delta w PSS (Kundur)  204/1, "MB-PSS 204 "/1  "<Rotor speed deviation  dw (pu)>"
  Real-Imag to Complex/1 -> Complex to Magnitude-Angle/1
  Complex to Magnitude-Angle/1 -> AC4A Excitation System 204/2, [Vt204]
  AC4A Excitation System 204/1 -> 204/2, [EFD204]
  Bus Selector1/5 -> [theta204]  "<Rotor mechanical angle  theta (deg)>"
  Bus Selector1/2 -> [Pe204]  "<Output active power   Peo (pu)>"
  Bus Selector1/8 -> AC4A Excitation System 204/3  "<Field current  ifd (pu)>"
  Bus Selector1/9 -> [Q204]  "<Output reactive power  Qeo (pu)>"
  STG 204/4 -> 204/1, [Pm204]
  PSS model4/1 -> Sum2/2
  Sum2/1 -> Multiport Switch1/1
  [PSSmodel] -> Sum2/1
  PSS model3/1 -> Multiport Switch1/2
  Sum3/1 -> [Pa204], "Delta Pa PSS 204 "/1  "Pm-Pe"
  "Delta Pa PSS 204 "/1 -> Multiport Switch1/5
  Delta w PSS (Kundur)  204/1 -> Multiport Switch1/4
  [Pm204] -> Sum3/2
  [Pe204] -> Sum3/1
  "MB-PSS 204 "/1 -> Multiport Switch1/3
  STG 204/1 -> Terminator3/1
  STG 204/2 -> Terminator1/1
  STG 204/3 -> Terminator2/1
  Pref1/1 -> STG 204/2
  Multiport Switch1/1 -> AC4A Excitation System 204/4, Scope4/1, [pss204]
  connections:
  204/RConn1 -- A/RConn1
  204/RConn2 -- B/RConn1
  204/RConn3 -- C/RConn1
